simulink model "motor_tuning"  (R2021a)
settings: Solver=FixedStepAuto  StartTime=0.0  StopTime=100.0  RelTol=1e-3  EnableMultiTasking=on
libraries: arduinolib x3
settings Model: SILPILModeSetting=veronly  ExtModeTrigDuration=2  Creator=admin  LastModifiedBy=admin
settings SolverCC: AutoInsertRateTranBlk=on
settings OptimizationCC: EnhancedBackFolding=on  PassReuseOutputArgsAs=Individual arguments  ZeroExternalMemoryAtStartup=off  ZeroInternalMemoryAtStartup=off  MaxStackSize=64  OptimizeBlockOrder=speed  DifferentSizesBufferReuse=on  OptimizationCustomize=off  EfficientTunableParamExpr=on
settings DebuggingCC: ParameterTunabilityLossMsg=error
settings HardwareCC: ProdBitPerPointer=32  ProdBitPerSizeT=32  ProdBitPerPtrDiffT=32  ProdLargestAtomicInteger=Long  ProdLargestAtomicFloat=Double  ProdWordSize=32  ProdHWDeviceType=ARM Compatible->ARM Cortex
settings SFSimCC: MATLABDynamicMemAlloc=off
settings RTWCC: SystemTargetFile=ert.tlc  HardwareBoard=Arduino Due  TemplateMakefile=ert_default_tmf  Toolchain=Arduino ARM  BuildConfiguration=Faster Runs
settings CodeAppCC: ForceParamTrailComments=on  IgnoreCustomStorageClasses=off  OperatorAnnotations=on  SimulinkDataObjDesc=on  SFDataObjDesc=on  InsertBlockDesc=on
settings ERTTargetCC: SupportContinuousTime=on  SupportVariableSizeSignals=on  ExtModeTransport=3  ExtModeStaticAlloc=on  ExtModeStaticAllocSize=24576  ExtModeMexFile=ext_xcp  ExtModeIntrfLevel=Level2 - Open

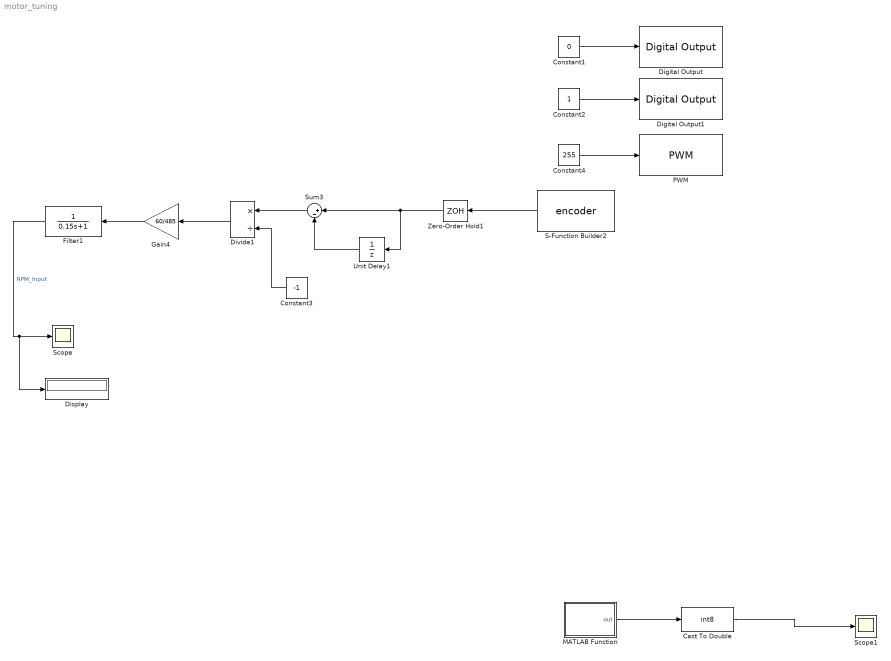
== system motor_tuning ==
  Cast To Double : DataTypeConversion  OutDataTypeStr=int8
  Constant1 : Constant  Value=0
  Constant2 : Constant
  Constant3 : Constant  Value=-1  VectorParams1D=off  SampleTime=-1
  Constant4 : Constant  Value=255
  Digital Output : arduinolib/Digital Output  pinNumber=5  Direction=output  blockPlatform=arduino
  Digital Output1 : arduinolib/Digital Output  pinNumber=6  Direction=output  blockPlatform=arduino
  Display : Display
  Divide1 : Product  Inputs=*/
  Filter1 : TransferFcn  Numerator=1  Denominator=[0.15 1]
  Gain4 : Gain  Gain=60/485
  MATLAB Function : MATLAB Function  TreatAsAtomicUnit=on
  PWM : arduinolib/PWM  pinNumber=4  frequencyType=Default  desiredFrequency=490.2  achievableFrequency=490.2
  S-Function Builder2 : S-Function  InitFcn=try, set_param(gcb,'FunctionName','encoder'), end  FunctionName=encoder  Parameters=int8(0),int8(2),int8(3)  SFunctionModules=encoder_wrapper  SFunctionDeploymentMode=off  EnableBusSupport=off  mask(S-Function Builder){}
      mask help: Simulink:masks:SFunctionBuilder_MD
      mask init:
      | val = [[.9  0.75 0.75 1 1 .9 .9 1]',[1 1 0.75 0.75 .9 .9 1 .9]'];try , sys = get_param(gcb,'SfunBuilderFcnName');if isempty(sys), sys = get_param(gcb,'FunctionName'); end,catch, sys = get_param(gcb,'FunctionName'); end
      settings: CopyFcn=set_param(gcbh,'LinkStatus','none')  PreSaveFcn=try, set_param(gcb,'FunctionName','encoder'), end  OpenFcn=sfunctionwizard(gcbh)
      mask Display: plot(val(:,1),val(:,2)),disp(sys), port_label('output',1,'pos')
  Scope : Scope
  Scope1 : Scope
  Sum3 : Sum  Inputs=|+-
  Unit Delay1 : UnitDelay  SampleTime=-1  HasFrameUpgradeWarning=on
  Zero-Order Hold1 : ZeroOrderHold  SampleTime=-1
  wires:
  Constant1/1 -> Digital Output/1
  Constant2/1 -> Digital Output1/1
  Gain4/1 -> Filter1/1
  Divide1/1 -> Gain4/1
  Sum3/1 -> Divide1/1
  Filter1/1 -> Display/1, Scope/1  "RPM_Input"
  Zero-Order Hold1/1 -> Sum3/1, Unit Delay1/1
  Constant3/1 -> Divide1/2
  S-Function Builder2/1 -> Zero-Order Hold1/1
  Unit Delay1/1 -> Sum3/2
  Constant4/1 -> PWM/1
  Cast To Double/1 -> Scope1/1
  MATLAB Function/1(out) -> Cast To Double/1

== matlab function motor_tuning/MATLAB Function ==
  data: out output
function out = fcn()
x = arduino('COM5','Due','Libraries','rotaryEncoder');
p = rotaryEncoder(x,'A0','A1',7);
y = readSpeed(p);
out = y;
